simulink model "TFBlock"  (R2014b)
settings: Solver=ode45  StartTime=0.0  StopTime=10.0  RelTol=1e-3
settings Model: Creator=99641  LastModifiedBy=99641

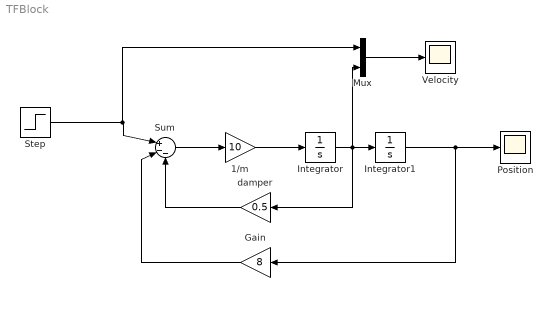
== system TFBlock ==
  1/m : Gain  Gain=10
  Gain : Gain  Gain=8
  Integrator : Integrator
  Integrator1 : Integrator
  Mux : Mux  Inputs=2
  Position : Scope
  Step : Step  SampleTime=0
  Sum : Sum  Inputs=|+--
  "Velocity " : Scope
  damper : Gain  Gain=0.5
  wires:
  1/m/1 -> Integrator/1
  Sum/1 -> 1/m/1
  Integrator/1 -> Mux/2, damper/1, Integrator1/1
  Integrator1/1 -> Gain/1, Position/1
  damper/1 -> Sum/3
  Gain/1 -> Sum/2
  Step/1 -> Mux/1, Sum/1
  Mux/1 -> "Velocity "/1
